simulink model "merge_test2"  (R2017b)
settings: Solver=FixedStepAuto  StartTime=0.0  StopTime=10.0  FixedStep=0.1  RelTol=1e-3  EnableMultiTasking=on
settings Model: Creator=hamza  LastModifiedBy=hbourbou
settings DataIOCC: SaveFormat=StructureWithTime
settings OptimizationCC: LifeSpan=inf
settings DebuggingCC: SFUnexpectedBacktrackingDiag=warning  SFNoUnconditionalDefaultTransitionDiag=warning  SFExecutionAtInitializationDiag=none
settings HardwareCC: ProdBitPerSizeT=32  ProdBitPerPtrDiffT=32  ProdWordSize=32  ProdHWDeviceType=Specified
settings CodeAppCC: StateflowObjectComments=on
settings GRTTargetCC: TargetLangStandard=C89/C90 (ANSI)  GeneratePreprocessorConditionals=Disable all
settings ConfigComp: CovMetricSettings=dw  CovHtmlReporting=on  CovSaveCumulativeToWorkspaceVar=on  CovSaveSingleToWorkspaceVar=on  CovExternalEMLEnable=off

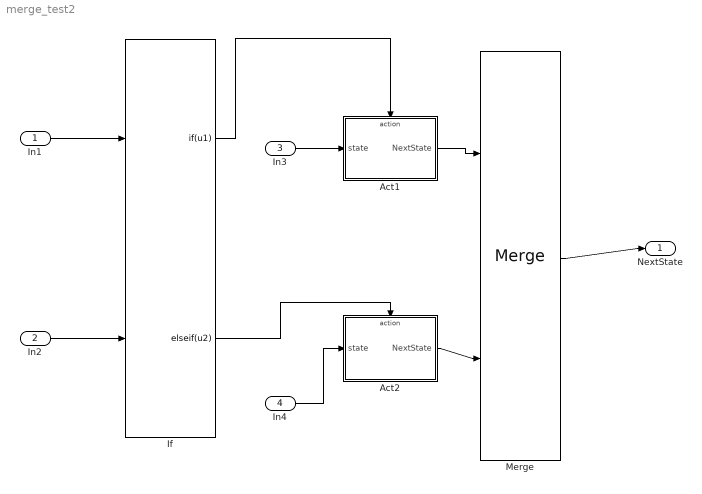
== system merge_test2 ==
  In1 : Inport  OutDataTypeStr=boolean
  In2 : Inport  Port=2  OutDataTypeStr=boolean
  In3 : Inport  Port=3  OutDataTypeStr=int16
  In4 : Inport  Port=4  OutDataTypeStr=int16
  Act1 : Subsystem
  Act2 : Subsystem
  If : If  NumInputs=2  IfExpression=u1  ElseIfExpressions=u2  ShowElse=off
  Merge : Merge
  NextState : Outport
  wires:
  In1/1 -> If/1
  If/1 -> Act1/Action
  In2/1 -> If/2
  If/2 -> Act2/Action
  In3/1 -> Act1/1(state)
  Act1/1(NextState) -> Merge/1
  Act2/1(NextState) -> Merge/2
  Merge/1 -> NextState/1
  In4/1 -> Act2/1(state)

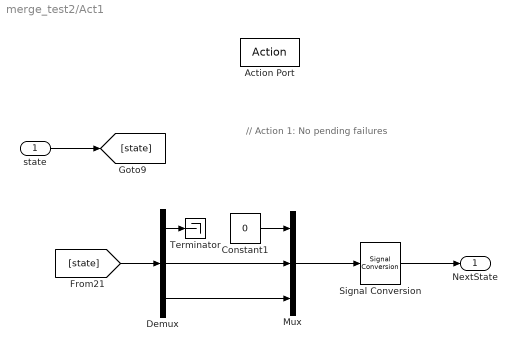
== system merge_test2/Act1 ==
  note: // Action 1: No pending failures
  state : Inport
  Action Port : ActionPort  ActionType=then
  Constant1 : Constant  Value=0  OutDataTypeStr=int16
  Demux : Demux  Outputs=3
  Mux : Mux  Inputs=3
  Signal Conversion : SignalConversion  OverrideOpt=off
  Terminator : Terminator
  NextState : Outport
  wires:
  state/1 -> [state]
  Signal Conversion/1 -> NextState/1
  Mux/1 -> Signal Conversion/1
  [state] -> Demux/1
  Demux/2 -> Mux/2
  Demux/3 -> Mux/3
  Constant1/1 -> Mux/1
  Demux/1 -> Terminator/1

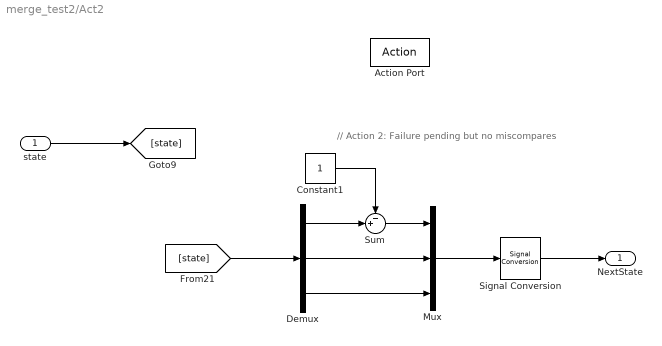
== system merge_test2/Act2 ==
  note: // Action 2: Failure pending but no miscompares
  state : Inport
  Action Port : ActionPort  ActionType=elseif
  Constant1 : Constant  OutDataTypeStr=int16
  Demux : Demux  Outputs=3
  Mux : Mux  Inputs=3
  Signal Conversion : SignalConversion  OverrideOpt=off
  Sum : Sum  Inputs=-+|
  NextState : Outport
  wires:
  state/1 -> [state]
  Constant1/1 -> Sum/1
  Signal Conversion/1 -> NextState/1
  Mux/1 -> Signal Conversion/1
  [state] -> Demux/1
  Demux/2 -> Mux/2
  Demux/3 -> Mux/3
  Sum/1 -> Mux/1
  Demux/1 -> Sum/2
